simulink model "adaptable_1c"  (Simulink 5.0)
settings: Solver=ode45  StartTime=0.0  StopTime=50  RelTol=1e-3
undefined symbols (not defined in the file): A, B, Blockset_Practica2, Diseño, ts
libraries: simulink x6, dsparch4 x2, dspstat3 x2
settings Model: LastModifiedBy=pc1

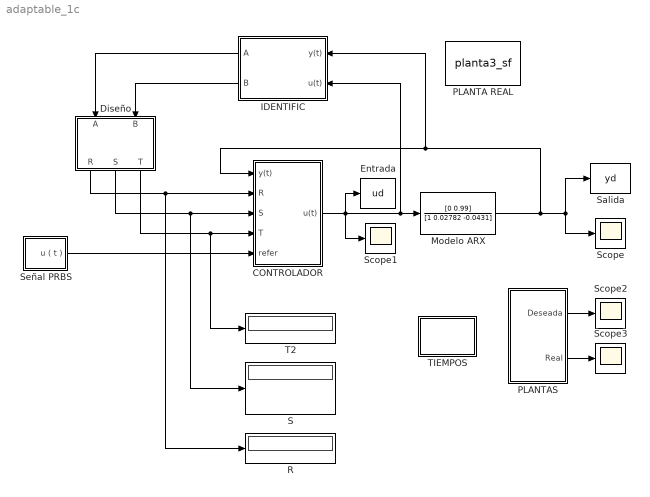
== system adaptable_1c ==
  CONTROLADOR : Subsystem
  Diseño : Subsystem  Orientation=down  AncestorBlock=Blockset_Practica2/Diseño  mask{Am=[1 -1.5489 .6], A0=1}
      mask Display: disp('Diseño')
  Entrada : ToWorkspace  VariableName=ud  SampleTime=-1  SaveFormat=Array
  IDENTIFIC : Subsystem  Orientation=left
  Modelo ARX : DiscreteFilter  Numerator=[0 0.99]  Denominator=[1 0.02782 -0.0431]  SampleTime=ts
  PLANTA REAL : S-Function  FunctionName=planta3_sf
  PLANTAS : Subsystem
  R : Display
  S : Display
  Salida : ToWorkspace  VariableName=yd  SampleTime=-1  SaveFormat=Array
  Scope{,1..3} (4 alike) : Scope
      Scope settings: TimeRange=10  YMin=0  YMax=1.4
      Scope1 settings: TimeRange=10  YMin=0  YMax=1.4  SaveName=ScopeData2
      Scope2 settings: TimeRange=10  YMin=0  YMax=1.4
      Scope3 settings: TimeRange=10  YMin=0  YMax=1.4  SaveName=ScopeData3
  Señal PRBS : Subsystem
  T2 : Display
  TIEMPOS : Subsystem
  wires:
  Modelo ARX/1 -> Scope/1, Salida/1, CONTROLADOR/1(y(t)), IDENTIFIC/1(y(t))
  CONTROLADOR/1(u(t)) -> Scope1/1, Entrada/1, IDENTIFIC/2(u(t)), Modelo ARX/1
  PLANTAS/1(Deseada) -> Scope2/1
  PLANTAS/2(Real) -> Scope3/1
  Diseño/1(R) -> CONTROLADOR/2(R), R/1
  Diseño/2(S) -> CONTROLADOR/3(S), S/1
  Diseño/3(T) -> CONTROLADOR/4(T), T2/1
  Señal PRBS/1(u ( t )) -> CONTROLADOR/5(refer)
  IDENTIFIC/2(B) -> Diseño/2(B)
  IDENTIFIC/1(A) -> Diseño/1(A)

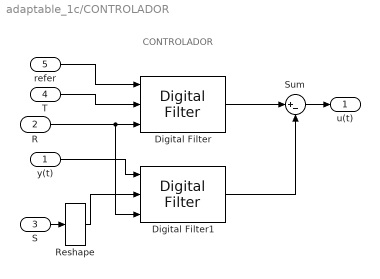
== system adaptable_1c/CONTROLADOR ==
  note: CONTROLADOR
  y(t) : Inport
  R : Inport  Port=2
  S : Inport  Port=3
  T : Inport  Port=4
  refer : Inport  Port=5
  Digital Filter : dsparch4/Digital Filter  TypePopup=IIR (poles & zeros)  IIRFiltStruct=Direct form II  AllPoleFiltStruct=Direct form  FIRFiltStruct=Direct form  CoeffSource=Input port(s)  NumCoeffs=[1 2]  DenCoeffs=[1 0.1]  BiQuadCoeffs=[1 0.3 0.4 1 0.1 0.2]  LatticeCoeffs=[0.2 0.4]  denIgnore=on  FiltPerSampPopup=One filter per frame  IC=0  ICnum=0  ICden=0
  Digital Filter1 : dsparch4/Digital Filter  TypePopup=IIR (poles & zeros)  IIRFiltStruct=Direct form II  AllPoleFiltStruct=Direct form  FIRFiltStruct=Direct form  CoeffSource=Input port(s)  NumCoeffs=[1 2]  DenCoeffs=[1 0.1]  BiQuadCoeffs=[1 0.3 0.4 1 0.1 0.2]  LatticeCoeffs=[0.2 0.4]  denIgnore=on  FiltPerSampPopup=One filter per frame  IC=0  ICnum=0  ICden=0
  Reshape : simulink/Math Operations/Reshape  OutputDimensionality=Column vector  OutputDimensions=[1,1]
  Sum : Sum  Inputs=|+-  SaturateOnIntegerOverflow=on
  u(t) : Outport
  wires:
  Sum/1 -> u(t)/1
  Digital Filter/1 -> Sum/1
  Digital Filter1/1 -> Sum/2
  y(t)/1 -> Digital Filter1/1
  R/1 -> Digital Filter1/3, Digital Filter/3
  Reshape/1 -> Digital Filter1/2
  T/1 -> Digital Filter/2
  refer/1 -> Digital Filter/1
  S/1 -> Reshape/1

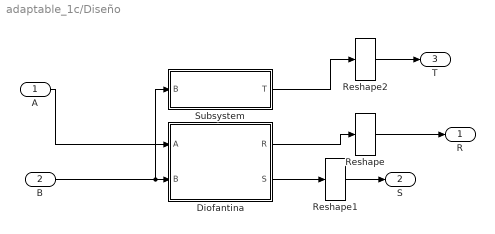
== system adaptable_1c/Diseño ==
  A : Inport
  B : Inport  Port=2
  Diofantina : Subsystem  mask{Ac=conv(Am,A0)}
      mask Display: disp('Diofantica')
  Reshape : simulink/Math Operations/Reshape  OutputDimensionality=Column vector  OutputDimensions=[1,1]
  Reshape1 : simulink/Math Operations/Reshape  OutputDimensionality=Column vector  OutputDimensions=[1,1]
  Reshape2 : simulink/Math Operations/Reshape  OutputDimensionality=Column vector  OutputDimensions=[1,1]
  Subsystem : Subsystem  mask{Am=Am, A0=A0}
      mask Display: disp('Polinomio T')
  R : Outport
  S : Outport  Port=2
  T : Outport  Port=3
  wires:
  Subsystem/1(T) -> Reshape2/1
  Diofantina/1(R) -> Reshape/1
  A/1 -> Diofantina/1(A)
  Diofantina/2(S) -> Reshape1/1
  B/1 -> Diofantina/2(B), Subsystem/1(B)
  Reshape/1 -> R/1
  Reshape1/1 -> S/1
  Reshape2/1 -> T/1

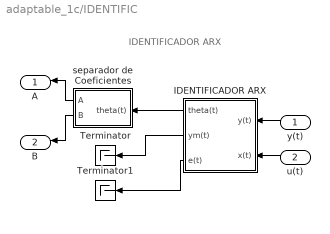
== system adaptable_1c/IDENTIFIC ==
  note: IDENTIFICADOR ARX
  y(t) : Inport  Orientation=left
  u(t) : Inport  Orientation=left  Port=2
  IDENTIFICADOR ARX : Subsystem  Orientation=left  mask{l=1, ts=ts, nk=1, nb=1, na=2}
      mask prompts: l "valor landa"; ts "valor ts"; nk "valor nk"; nb "valor nb"; na "Valor na"
  Terminator : Terminator
  Terminator1 : Terminator
  separador de Coeficientes : Subsystem  Orientation=left  mask{na=2, nb=1}
  A : Outport  Orientation=left
  B : Outport  Orientation=left  Port=2
  wires:
  IDENTIFICADOR ARX/1(theta(t)) -> separador de Coeficientes/1(theta(t))
  IDENTIFICADOR ARX/2(ym(t)) -> Terminator/1
  IDENTIFICADOR ARX/3(e(t)) -> Terminator1/1
  separador de Coeficientes/1(A) -> A/1
  separador de Coeficientes/2(B) -> B/1
  y(t)/1 -> IDENTIFICADOR ARX/1(y(t))
  u(t)/1 -> IDENTIFICADOR ARX/2(x(t))

== system adaptable_1c/PLANTAS ==
  PLANT REAL : S-Function  FunctionName=planta3_sf
  Planta Deseada : Subsystem  mask{Bm=[1]*.05105, Am=[1 -1.5489 .6], ts=ts}
      mask prompts: Bm "Polinomio Numerador Bm"; Am "Polinomio Denominador Am"; ts "Tiempo de Muestreo"
  Step1 : Step  Time=0  SampleTime=0
  Deseada : Outport
  Real : Outport  Port=2
  wires:
  Step1/1 -> Planta Deseada/1(u(t)), PLANT REAL/1
  Planta Deseada/1(y(t)) -> Deseada/1
  PLANT REAL/1 -> Real/1

== system adaptable_1c/Señal PRBS ==
  Random Number : RandomNumber  Variance=.001  SampleTime=0
  Sign : Signum
  Zero-Order Hold : ZeroOrderHold  SampleTime=.1
  u ( t ) : Outport
  wires:
  Zero-Order Hold/1 -> u ( t )/1
  Sign/1 -> Zero-Order Hold/1
  Random Number/1 -> Sign/1

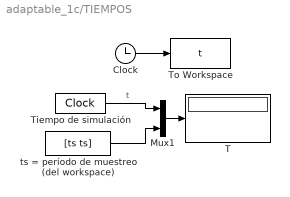
== system adaptable_1c/TIEMPOS ==
  Clock : Clock
      settings: Decimation=10
  Mux1 : Mux  Inputs=2
  T : Display
  Tiempo de simulación : DigitalClock  SampleTime=.1
  To Workspace : ToWorkspace  VariableName=t  SampleTime=ts  SaveFormat=Array
  ts = período de muestreo (del workspace) : FromWorkspace  VariableName=[ts ts]  SampleTime=0
  wires:
  Clock/1 -> To Workspace/1
  ts = período de muestreo (del workspace)/1 -> Mux1/2
  Tiempo de simulación/1 -> Mux1/1  "t"
  Mux1/1 -> T/1

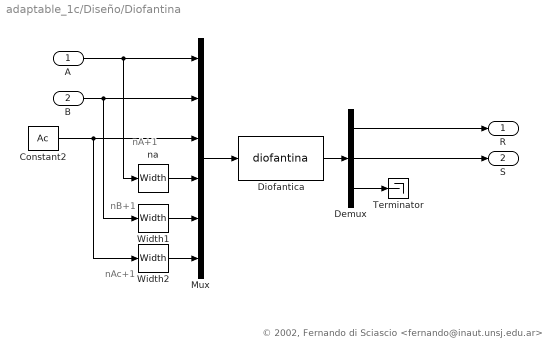
== system adaptable_1c/Diseño/Diofantina ==
  note: nAc+1
  note: nA+1
  note: nB+1
  note: © 2002, Fernando di Sciascio <fernando@inaut.unsj.edu.ar>
  A : Inport
  B : Inport  Port=2
  Constant2 : Constant  Value=Ac
  Demux : Demux  Outputs="[length(Ac)-length(A)+1  length(A)-1  length(A)+length(B)+length(Ac) - (length(Ac)-length(A)+1) -  ( length(A)-1 )+3]"
  Diofantica : S-Function  FunctionName=diofantina
      mask Type: S-function: timestwo
      mask Description: Esta S-function resuelve la ecuacion diofantina
      mask Help:
      | Dados los polinomios A, B, Ac y los ordenes de los polinomios R y S esta
      | S-function resuelve la ecuacion diofantina:
      | 
      |     A*R+B*S=Ac
      mask Display: disp('        Diofantina      ');
  Mux : Mux  Inputs=6
  Terminator : Terminator
  Width1 : Width
  Width2 : Width
  na : Width
  R : Outport
  S : Outport  Port=2
  wires:
  Mux/1 -> Diofantica/1
  Constant2/1 -> Mux/3, Width2/1
  Diofantica/1 -> Demux/1
  Demux/3 -> Terminator/1
  A/1 -> Mux/1, na/1
  B/1 -> Mux/2, Width1/1
  Demux/1 -> R/1
  Demux/2 -> S/1
  na/1 -> Mux/4
  Width1/1 -> Mux/5
  Width2/1 -> Mux/6

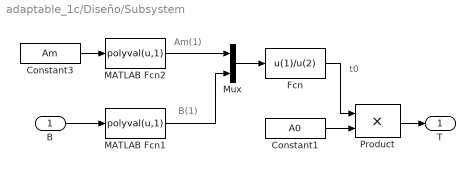
== system adaptable_1c/Diseño/Subsystem ==
  note: B(1)
  note: Am(1)
  note: t0
  B : Inport
  Constant1 : Constant  Value=A0
  Constant3 : Constant  Value=Am
  Fcn : Fcn  Expr=u(1)/u(2)
  MATLAB Fcn1 : MATLABFcn  MATLABFcn=polyval(u,1)
  MATLAB Fcn2 : MATLABFcn  MATLABFcn=polyval(u,1)
  Mux : Mux  Inputs=2
  Product : Product  SaturateOnIntegerOverflow=on  InputSameDT=on
  T : Outport
  wires:
  Mux/1 -> Fcn/1
  MATLAB Fcn2/1 -> Mux/1
  MATLAB Fcn1/1 -> Mux/2
  Fcn/1 -> Product/1
  Constant3/1 -> MATLAB Fcn2/1
  Product/1 -> T/1
  B/1 -> MATLAB Fcn1/1
  Constant1/1 -> Product/2

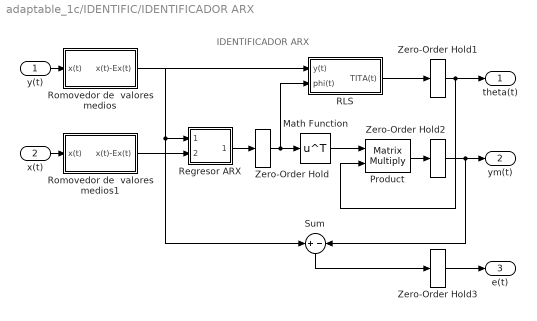
== system adaptable_1c/IDENTIFIC/IDENTIFICADOR ARX ==
  note: IDENTIFICADOR ARX
  y(t) : Inport
  x(t) : Inport  Port=2
  Math Function : Math  Operator=transpose
  Product : Product  Multiplication=Matrix(*)  SaturateOnIntegerOverflow=on  InputSameDT=on
  RLS : Subsystem
  Regresor ARX : Subsystem
  Romovedor de  valores medios : Subsystem
  Romovedor de  valores medios1 : Subsystem
  Sum : Sum  Orientation=down  Inputs=+-  SaturateOnIntegerOverflow=on  InputSameDT=on
  Zero-Order Hold{,1..3} (4 alike) : ZeroOrderHold  SampleTime=ts
  theta(t) : Outport
  ym(t) : Outport  Port=2
  e(t) : Outport  Port=3
  wires:
  Math Function/1 -> Product/1
  Zero-Order Hold3/1 -> e(t)/1
  Product/1 -> Zero-Order Hold2/1
  Zero-Order Hold1/1 -> theta(t)/1, Product/2
  Zero-Order Hold/1 -> RLS/2(phi(t)), Math Function/1
  RLS/1(TITA(t)) -> Zero-Order Hold1/1
  x(t)/1 -> Romovedor de  valores medios1/1(x(t))
  y(t)/1 -> Romovedor de  valores medios/1(x(t))
  Romovedor de  valores medios/1(x(t)-Ex(t)) -> RLS/1(y(t)), Regresor ARX/1(y(t)), Sum/1
  Romovedor de  valores medios1/1(x(t)-Ex(t)) -> Regresor ARX/2(u(t))
  Regresor ARX/1(phi) -> Zero-Order Hold/1
  Zero-Order Hold2/1 -> ym(t)/1, Sum/2
  Sum/1 -> Zero-Order Hold3/1

== system adaptable_1c/IDENTIFIC/separador de Coeficientes ==
  theta(t) : Inport
  Demux : Demux  Outputs=[na,nb]
  A : Outport
  B : Outport  Port=2
  wires:
  Demux/1 -> A/1
  theta(t)/1 -> Demux/1
  Demux/2 -> B/1

== system adaptable_1c/PLANTAS/Planta Deseada ==
  u(t) : Inport
  Discrete Transfer Fcn : DiscreteTransferFcn  Numerator=Bm  Denominator=Am  SampleTime=ts
  y(t) : Outport
  wires:
  u(t)/1 -> Discrete Transfer Fcn/1
  Discrete Transfer Fcn/1 -> y(t)/1

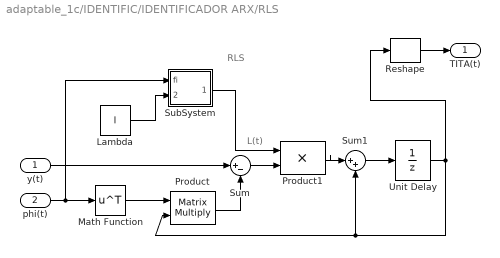
== system adaptable_1c/IDENTIFIC/IDENTIFICADOR ARX/RLS ==
  note: RLS
  note: L(t)
  y(t) : Inport
  phi(t) : Inport  Port=2
  Lambda : Constant  Value=l
  Math Function : Math  Operator=transpose
  Product : Product  Multiplication=Matrix(*)  SaturateOnIntegerOverflow=on  InputSameDT=on
  Product1 : Product  SaturateOnIntegerOverflow=on  InputSameDT=on
  Reshape : simulink/Math Operations/Reshape  OutputDimensionality=Column vector  OutputDimensions=[1,1]
  SubSystem : Subsystem
  Sum : Sum  Inputs=|+-  SaturateOnIntegerOverflow=on  InputSameDT=on
  Sum1 : Sum  Inputs=|++  SaturateOnIntegerOverflow=on  InputSameDT=on
  Unit Delay : UnitDelay  X0=zeros(1,na+nb)'  SampleTime=ts
  TITA(t) : Outport
  wires:
  phi(t)/1 -> SubSystem/1(fi), Math Function/1
  Math Function/1 -> Product/1
  Unit Delay/1 -> Product/2, Sum1/2, Reshape/1
  Product/1 -> Sum/2
  y(t)/1 -> Sum/1
  Sum/1 -> Product1/2
  SubSystem/1(L(t)) -> Product1/1
  Lambda/1 -> SubSystem/2(landa)
  Sum1/1 -> Unit Delay/1
  Product1/1 -> Sum1/1
  Reshape/1 -> TITA(t)/1

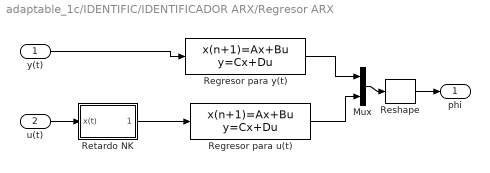
== system adaptable_1c/IDENTIFIC/IDENTIFICADOR ARX/Regresor ARX ==
  y(t) : Inport
  u(t) : Inport  Port=2
  Mux : Mux  Inputs=2
  Regresor para u(t) : DiscreteStateSpace  A=[zeros(1,nb);eye(nb-1,nb)]  B=[1,zeros(1,nb-1)]'  C=eye(nb)  D=[zeros(nb,1)]  SampleTime=ts
  Regresor para y(t) : DiscreteStateSpace  A=[zeros(1,na);eye(na-1,na)]  B=[-1,zeros(1,na-1)]'  C=eye(na)  D=[zeros(na,1)]  SampleTime=ts
  Reshape : simulink/Math Operations/Reshape  OutputDimensionality=Column vector  OutputDimensions=[1,1]
  Retardo NK : Subsystem  mask{nk=nk}
      mask prompts: nk "Valor nk"
  phi : Outport
  wires:
  Reshape/1 -> phi/1
  Retardo NK/1(x(t-nk)) -> Regresor para u(t)/1
  u(t)/1 -> Retardo NK/1(x(t))
  Mux/1 -> Reshape/1
  y(t)/1 -> Regresor para y(t)/1
  Regresor para u(t)/1 -> Mux/2
  Regresor para y(t)/1 -> Mux/1

== system adaptable_1c/IDENTIFIC/IDENTIFICADOR ARX/Romovedor de  valores medios ==
  x(t) : Inport
  Mean : dspstat3/Mean  run=on  reset_popup=None
  Sum : Sum  Inputs=|-+  SaturateOnIntegerOverflow=on  InputSameDT=on
  Zero-Order Hold : ZeroOrderHold  SampleTime=ts
  x(t)-Ex(t) : Outport
  wires:
  x(t)/1 -> Zero-Order Hold/1
  Zero-Order Hold/1 -> Mean/1, Sum/2
  Mean/1 -> Sum/1
  Sum/1 -> x(t)-Ex(t)/1

== system adaptable_1c/IDENTIFIC/IDENTIFICADOR ARX/Romovedor de  valores medios1 ==
  x(t) : Inport
  Mean : dspstat3/Mean  run=on  reset_popup=None
  Sum : Sum  Inputs=|-+  SaturateOnIntegerOverflow=on  InputSameDT=on
  Zero-Order Hold : ZeroOrderHold  SampleTime=ts
  x(t)-Ex(t) : Outport
  wires:
  x(t)/1 -> Zero-Order Hold/1
  Zero-Order Hold/1 -> Mean/1, Sum/2
  Mean/1 -> Sum/1
  Sum/1 -> x(t)-Ex(t)/1

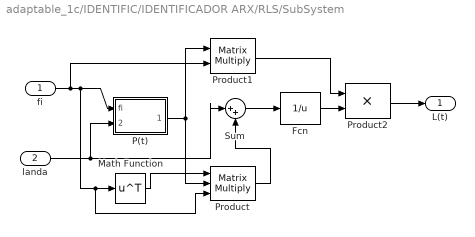
== system adaptable_1c/IDENTIFIC/IDENTIFICADOR ARX/RLS/SubSystem ==
  fi : Inport
  landa : Inport  Port=2
  Fcn : Fcn  Expr=1/u
  Math Function : Math  Operator=transpose
  P(t) : Subsystem
  Product : Product  Inputs=3  Multiplication=Matrix(*)  SaturateOnIntegerOverflow=on  InputSameDT=on
  Product1 : Product  Multiplication=Matrix(*)  SaturateOnIntegerOverflow=on  InputSameDT=on
  Product2 : Product  SaturateOnIntegerOverflow=on  InputSameDT=on
  Sum : Sum  Inputs=|++  SaturateOnIntegerOverflow=on  InputSameDT=on
  L(t) : Outport
  wires:
  Product2/1 -> L(t)/1
  P(t)/1(P(t-1)) -> Product/2, Product1/1
  fi/1 -> P(t)/1(fi), Math Function/1, Product/3, Product1/2
  landa/1 -> P(t)/2(landa), Sum/1
  Math Function/1 -> Product/1
  Product/1 -> Sum/2
  Sum/1 -> Fcn/1
  Fcn/1 -> Product2/2
  Product1/1 -> Product2/1

== system adaptable_1c/IDENTIFIC/IDENTIFICADOR ARX/Regresor ARX/Retardo NK ==
  x(t) : Inport
  Constant : Constant  Value=nk
  Multiport Switch2 : MultiPortSwitch  Inputs=2  SaturateOnIntegerOverflow=on  InputSameDT=on
  Retraso nk : DiscreteStateSpace  A=[zeros(1,max(nk,1));eye(max(nk,1)-1,max(nk,1))]  B=[1,zeros(1,max(nk,1)-1)]'  C=[zeros(1,max(nk,1)-1),1]  D=[0]  SampleTime=ts
  Saturation : Saturate  UpperLimit=2  LowerLimit=0
  x(t-nk) : Outport
  wires:
  x(t)/1 -> Retraso nk/1, Multiport Switch2/2
  Multiport Switch2/1 -> x(t-nk)/1
  Retraso nk/1 -> Multiport Switch2/3
  Constant/1 -> Saturation/1
  Saturation/1 -> Multiport Switch2/1

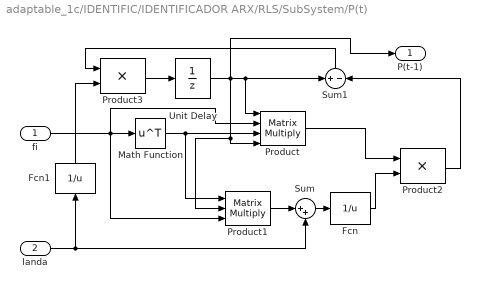
== system adaptable_1c/IDENTIFIC/IDENTIFICADOR ARX/RLS/SubSystem/P(t) ==
  fi : Inport
  landa : Inport  Port=2
  Fcn : Fcn  Expr=1/u
  Fcn1 : Fcn  Orientation=up  Expr=1/u
  Math Function : Math  Operator=transpose
  Product : Product  Inputs=4  Multiplication=Matrix(*)  SaturateOnIntegerOverflow=on  InputSameDT=on
  Product1 : Product  Inputs=3  Multiplication=Matrix(*)  SaturateOnIntegerOverflow=on  InputSameDT=on
  Product2 : Product  SaturateOnIntegerOverflow=on  InputSameDT=on
  Product3 : Product  SaturateOnIntegerOverflow=on  InputSameDT=on
  Sum : Sum  Inputs=|++  SaturateOnIntegerOverflow=on  InputSameDT=on
  Sum1 : Sum  Orientation=up  Inputs=+-  SaturateOnIntegerOverflow=on  InputSameDT=on
  Unit Delay : UnitDelay  X0=100000*eye(na+nb)  SampleTime=ts
  P(t-1) : Outport
  wires:
  Fcn1/1 -> Product3/2
  fi/1 -> Math Function/1, Product/2, Product1/3
  Unit Delay/1 -> P(t-1)/1, Product/4, Product1/2, Product/1, Sum1/1
  Math Function/1 -> Product/3, Product1/1
  Product1/1 -> Sum/1
  landa/1 -> Fcn1/1, Sum/2
  Sum/1 -> Fcn/1
  Fcn/1 -> Product2/2
  Product/1 -> Product2/1
  Sum1/1 -> Product3/1
  Product3/1 -> Unit Delay/1
  Product2/1 -> Sum1/2
